simulink model "PWM_Conversion"  (R2019b)
settings: Solver=VariableStepAuto  StartTime=0.0  StopTime=10.0  RelTol=1e-3
settings Model: Creator=spuny  LastModifiedBy=spuny

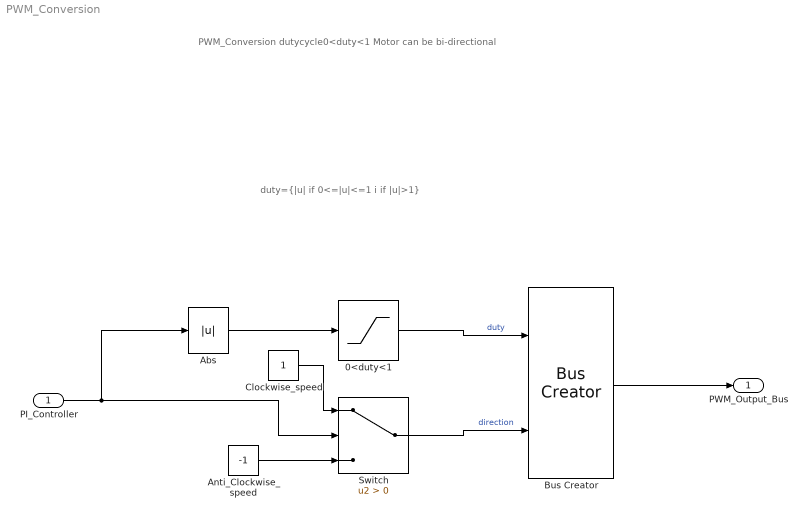
== system PWM_Conversion ==
  note: duty={|u| if 0<=|u|<=1
      | i if |u|>1}
  note: PWM_Conversion
      | dutycycle0<duty<1
      | Motor can be bi-directional
  "PI_Controller " : Inport
  "0<duty<1 " : Saturate
  Abs : Abs
  "Anti_Clockwise_speed " : Constant  Value=-1
  Bus Creator : BusCreator  Inputs=2  OutDataTypeStr=Bus: PWM_Output_Bus  NonVirtualBus=on
  "Clockwise_speed " : Constant
  Switch : Switch  Criteria=u2 > Threshold
  PWM_Output_Bus : Outport  OutDataTypeStr=Bus: PWM_Output_Bus
  wires:
  "PI_Controller "/1 -> Switch/2, Abs/1
  "Clockwise_speed "/1 -> Switch/1
  "Anti_Clockwise_speed "/1 -> Switch/3
  Switch/1 -> Bus Creator/2  "direction"
  Abs/1 -> "0<duty<1 "/1
  "0<duty<1 "/1 -> Bus Creator/1  "duty"
  Bus Creator/1 -> PWM_Output_Bus/1
